simulink model "position"  (R2022a)
settings: Solver=ode1  StartTime=0.0  StopTime=8  FixedStep=0.001  RelTol=1e-3  EnableMultiTasking=on
undefined symbols (not defined in the file): a, b, k1, k2
libraries: arduinolib x4, arduinosensorlib x1
settings Model: ExtModeTrigDuration=2  Creator=LabPC  LastModifiedBy=LabPC
settings SolverCC: AutoInsertRateTranBlk=on
settings OptimizationCC: EnhancedBackFolding=on  PassReuseOutputArgsAs=Individual arguments  ZeroExternalMemoryAtStartup=off  ZeroInternalMemoryAtStartup=off  MaxStackSize=64  OptimizeBlockOrder=speed  DifferentSizesBufferReuse=on  OptimizationCustomize=off  EfficientTunableParamExpr=on
settings DebuggingCC: ParameterTunabilityLossMsg=error
settings HardwareCC: ProdBitPerPointer=32  ProdBitPerSizeT=32  ProdBitPerPtrDiffT=32  ProdLargestAtomicInteger=Long  ProdLargestAtomicFloat=Double  ProdWordSize=32  ProdHWDeviceType=ARM Compatible->ARM Cortex
settings SFSimCC: MATLABDynamicMemAlloc=off
settings RTWCC: SystemTargetFile=ert.tlc  HardwareBoard=Arduino Due  TemplateMakefile=ert_default_tmf  Toolchain=Arduino ARM  BuildConfiguration=Faster Runs
settings CodeAppCC: ForceParamTrailComments=on  IgnoreCustomStorageClasses=off  OperatorAnnotations=on  SimulinkDataObjDesc=on  SFDataObjDesc=on  InsertBlockDesc=on
settings ERTTargetCC: SupportContinuousTime=on  SupportVariableSizeSignals=on  ExtModeTransport=3  ExtModeStaticAlloc=on  ExtModeStaticAllocSize=24576  ExtModeMexFile=ext_xcp  ExtModeIntrfLevel=Level2 - Open

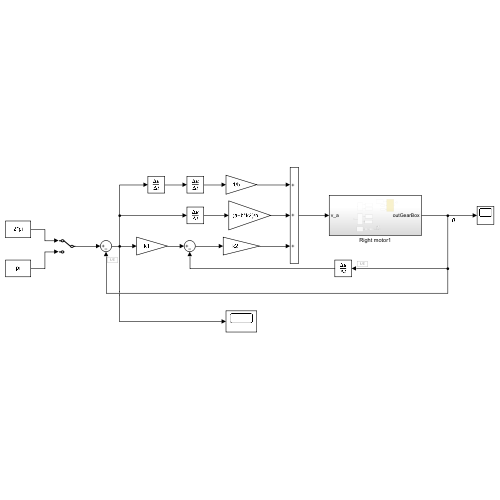
[thumbnail: Simulink's stored preview of the top-level diagram]
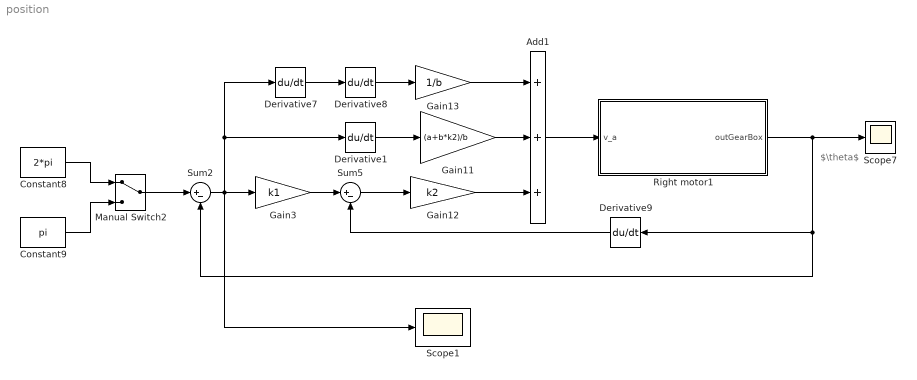
== system position ==
  note: $\theta$
  Add1 : Sum  Inputs=+++
  Constant8 : Constant  Value=2*pi
  Constant9 : Constant  Value=pi
  Derivative{1,7..9} (4 alike) : Derivative
  Gain11 : Gain  Gain=(a+b*k2)/b
  Gain12 : Gain  Gain=k2
  Gain13 : Gain  Gain=1/b
  Gain3 : Gain  Gain=k1
  Manual Switch2 : ManualSwitch
  Right motor1 : Subsystem
  Scope1 : Scope
  Scope7 : Scope
  Sum2 : Sum  Inputs=|+-
  Sum5 : Sum  Inputs=|+-
  wires:
  Right motor1/1(outGearBox) -> Sum2/2, Derivative9/1, Scope7/1
  Derivative8/1 -> Gain13/1
  Add1/1 -> Right motor1/1(v_a)
  Constant9/1 -> Manual Switch2/2
  Sum2/1 -> Scope1/1, Derivative7/1, Derivative1/1, Gain3/1
  Gain11/1 -> Add1/2
  Derivative9/1 -> Sum5/2
  Manual Switch2/1 -> Sum2/1
  Derivative1/1 -> Gain11/1
  Gain3/1 -> Sum5/1
  Constant8/1 -> Manual Switch2/1
  Gain13/1 -> Add1/1
  Derivative7/1 -> Derivative8/1
  Gain12/1 -> Add1/3
  Sum5/1 -> Gain12/1

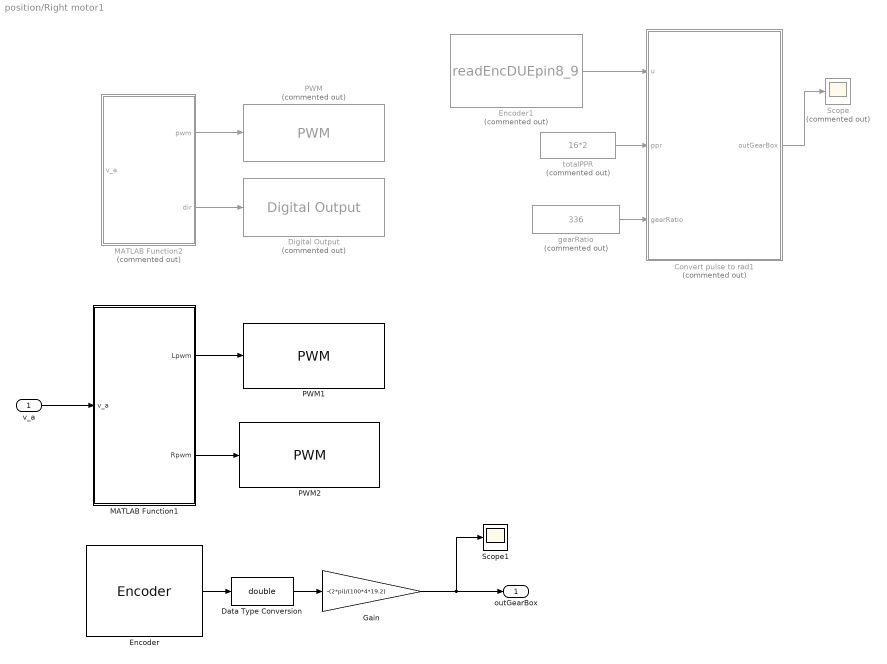
== system position/Right motor1 ==
  v_a : Inport
  Convert pulse to rad1 : MATLAB Function  Commented=on  TreatAsAtomicUnit=on
  Data Type Conversion : DataTypeConversion  OutDataTypeStr=double  SaturateOnIntegerOverflow=off  RndMeth=Floor
  Digital Output : arduinolib/Digital Output  Commented=on  pinNumber=7  Direction=output  blockPlatform=arduino
  Encoder : arduinosensorlib/Encoder  InputA=2  InputB=3  Mode=No reset  SampleTime=0.01
      settings: SourceProductBaseCode=ARDUINO
  Encoder1 : S-Function  Commented=on  InitFcn=try, set_param(gcb,'FunctionName','readEncDUEpin8_9'), end  FunctionName=readEncDUEpin8_9  SFunctionModules=readEncDUEpin8_9_wrapper  SFunctionDeploymentMode=off  EnableBusSupport=off  mask(S-Function Builder){}
      mask help: Simulink:masks:SFunctionBuilder_MD
      mask init:
      | val = [[.9  0.75 0.75 1 1 .9 .9 1]',[1 1 0.75 0.75 .9 .9 1 .9]'];try , sys = get_param(gcb,'SfunBuilderFcnName');if isempty(sys), sys = get_param(gcb,'FunctionName'); end,catch, sys = get_param(gcb,'FunctionName'); end
      settings: CopyFcn=set_param(gcbh,'LinkStatus','none')  PreSaveFcn=try, set_param(gcb,'FunctionName','readEncDUEpin8_9'), end  OpenFcn=sfunctionwizard(gcbh)
      mask Display:
      | plot(val(:,1),val(:,2))
      | disp(sys)
      | port_label('output',1,'count')
  Gain : Gain  Gain=-(2*pi)/(100*4*19.2)
  MATLAB Function1 : MATLAB Function  TreatAsAtomicUnit=on
  MATLAB Function2 : MATLAB Function  Commented=on  TreatAsAtomicUnit=on
  PWM : arduinolib/PWM  Commented=on  pinNumber=5  frequencyType=Default  desiredFrequency=490.2  achievableFrequency=490.2
  PWM1 : arduinolib/PWM  pinNumber=6  frequencyType=Default  desiredFrequency=490.2  achievableFrequency=490.2
  PWM2 : arduinolib/PWM  pinNumber=7  frequencyType=Default  desiredFrequency=490.2  achievableFrequency=490.2
  Scope : Scope  Commented=on
  Scope1 : Scope
  gearRatio : Constant  Commented=on  Value=336
  totalPPR : Constant  Commented=on  Value=16*2
  outGearBox : Outport
  wires:
  Gain/1 -> Scope1/1, outGearBox/1
  Encoder/1 -> Data Type Conversion/1
  v_a/1 -> MATLAB Function1/1(v_a)
  MATLAB Function1/2(Rpwm) -> PWM2/1
  MATLAB Function1/1(Lpwm) -> PWM1/1
  Encoder1/1 -> Convert pulse to rad1/1(u)
  Convert pulse to rad1/1(outGearBox) -> Scope/1
  gearRatio/1 -> Convert pulse to rad1/3(gearRatio)
  MATLAB Function2/1(pwm) -> PWM/1
  MATLAB Function2/2(dir) -> Digital Output/1
  totalPPR/1 -> Convert pulse to rad1/2(ppr)
  Data Type Conversion/1 -> Gain/1

== matlab function position/Right motor1/Convert pulse to rad1 ==
  settings: updateMethod=DISCRETE
  data: u input; ppr input; gearRatio input; outGearBox output
function outGearBox = fcn(u,ppr,gearRatio)

persistent counter_num over_flag
if(isempty(counter_num)), counter_num = 0;end
if(isempty(over_flag)), over_flag = 0;end
pulse2radian = 2*pi/ppr; % 1 pulse = ?? radian

if(double(u) - counter_num > 40000), over_flag = over_flag-1;
elseif(double(u) - counter_num < -40000), over_flag = over_flag+1;
end

inGearBox = (double(u)+over_flag*(2^32 -1))*pulse2radian; 
outGearBox = inGearBox/gearRatio;
counter_num = double(u) ;

== matlab function position/Right motor1/MATLAB Function1 ==
  data: v_a input; Lpwm output; Rpwm output
function [Lpwm,Rpwm] = fcn(v_a)

vmax = 22.9;
pwm_cal = v_a*254/vmax;

if pwm_cal > 0
    Lpwm = 0;
    Rpwm = pwm_cal;
elseif pwm_cal < 0
    Lpwm = abs(pwm_cal);
    Rpwm = 0;
else
    Lpwm = 0;
    Rpwm = 0;
end

== matlab function position/Right motor1/MATLAB Function2 ==
  data: v_a input; pwm output; dir output
function [pwm,dir] = fcn(v_a)

vmax = 22.9;
%vmax = 10;
pwm_cal = v_a*254/vmax;
if pwm_cal > 0
    pwm = pwm_cal;
    dir = 0;
elseif pwm_cal < 0
    pwm = abs(pwm_cal);
    dir = 1;
else
    pwm = 0;
    dir = 0;
end
